simulink model "mysldemo_2counters"  (R2014a)
settings: Solver=FixedStepDiscrete  StartTime=0.0  StopTime=2.5  FixedStep=.01  RelTol=1e-3  AbsTol=1e-6
undefined symbols (not defined in the file): sigbuilder_block
Description:
  | Counters Using Conditionally Executed Subsystems
  | 
  | This demonstration uses counter circuits to contrast the execution of blocks in enabled
  | subsystems and triggered subsystems for the same control signal. After running the
  | simulation, the scope shows three plots.
  | 
  | The first of these plots shows the control signal which is the output of the discrete
  | pulse generator.
  | 
  | The second plot shows the output of the counter circuit in the enabled subsystem.
  | The counter increments while the subsystem is enabled and then holds its output when
  | the subsystem is disabled. The counter resets to zero when the subsystem is re-enabled
  | because the enable port was configured to reset states when enabling.
  | 
  | The third plot shows the output of the counter circuit in the triggered subsystem. The
  | counter increments every rising edge of the control signal.
  | 
  | The signals are shown in a Signal Viewer scope that does not require a scope block to
  | be put into the block diagram.  Instead, the "glasses" icon notation on the ports show
  | that a Signal Viewer is attached.  Double click on the glasses to make the Signal
  | Viewer appear if it is hidden.
settings Model: RecordCoverage=on  CovMetricSettings=de  CovHTMLOptions=-aTS=1 -bRG=1 -bTC=1 -hTR=0 -nFC=0 -scm=1 -bcm=1 -xEv=0  CovHtmlReporting=off  CovForceBlockReductionOff=off  covSaveCumulativeToWorkspaceVar=off  CovSaveSingleToWorkspaceVar=off  CovCumulativeReport=on  CovReportOnPause=off  ExtModeTrigMode=oneshot  ExtModeArmWhenConnect=off  ExtModeAutoUpdateStatusClock=off  Creator=The MathWorks Inc.  LastModifiedBy=gxnuhuang
settings DataIOCC: LimitDataPoints=off  SaveFormat=StructureWithTime  DSMLogging=off  InspectSignalLogs=on  ReturnWorkspaceOutputs=on
settings OptimizationCC: BlockReduction=off  BooleanDataType=off  ExpressionDepthLimit=2147483647  InitFltsAndDblsToZero=on  BufferReusableBoundary=off
settings DebuggingCC: SaveWithParameterizedLinksMsg=none  UnderspecifiedInitializationDetection=Classic  SignalResolutionControl=TryResolveAllWithWarning  SolverPrmCheckMsg=none  MultiTaskDSMMsg=warning  MultiTaskCondExecSysMsg=none  FcnCallInpInsideContextMsg=UseLocalSettings  BusObjectLabelMismatch=none  StateNameClashWarn=warning
settings HardwareCC: TargetUnknown=on
settings RTWCC: IncludeERTFirstTime=on
settings GRTTargetCC: TargetFcnLib=ansi_tfl_tmw.mat  CombineOutputUpdateFcns=off  GRTInterface=on

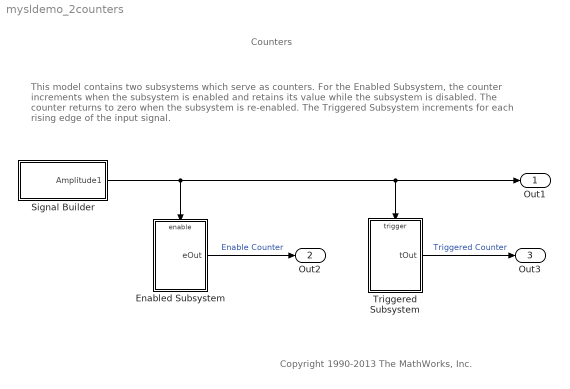
== system mysldemo_2counters ==
  note: Counters
  note: Copyright 1990-2013 The MathWorks, Inc.
  note: This model contains two subsystems which serve as counters. For the Enabled Subsystem, the counter
      | increments when the subsystem is enabled and retains its value while the subsystem is disabled.
      | The counter returns to zero when the subsystem is re-enabled.  The Triggered Subsystem increments
      | for each rising edge of the input signal.
  Enabled Subsystem : Subsystem  TreatAsAtomicUnit=on
  Signal Builder : Subsystem  Tag=STV Subsys  LoadFcn=sigbuilder_block('load');  StartFcn=sigbuilder_block('start');  StopFcn=sigbuilder_block('stop');  ClipboardFcn=sigbuilder_block('clipboard');  mask(Sigbuilder block){}
      mask help: Create and generate interchangeable groups of signals whose waveforms are piecewise linear.
      mask init:
      | if ~strcmp(get_param(bdroot(gcbh),'SimulationStatus'),'stopped') tuvar = sigbuilder_block('maskInit'); end
      settings: CopyFcn=sigbuilder_block('copy');  DeleteFcn=sigbuilder_block('delete');  ModelCloseFcn=sigbuilder_block('modelClose');  PreSaveFcn=sigbuilder_block('preSave');  PauseFcn=sigbuilder_block('pause')  ContinueFcn=sigbuilder_block('continue')  NameChangeFcn=sigbuilder_block('namechange');  OpenFcn=sigbuilder_block('open',[192.75 138 550.5 399.75 ]);  CloseFcn=sigbuilder_block('close');
      mask Display: plot(0,0,100,100,[10,10,40,40,10],[80,20,20,80,80],[40,10],[50,50], [40,27,10],[65,72,56],[40,25,25,10],[28,28,43,43]);
  Triggered Subsystem : Subsystem  TreatAsAtomicUnit=on
  Out1 : Outport
  Out2 : Outport  Port=2
  Out3 : Outport  Port=3
  wires:
  Enabled Subsystem/1(eOut) -> Out2/1  "Enable Counter"
  Triggered Subsystem/1(tOut) -> Out3/1  "Triggered Counter"
  Signal Builder/1(Amplitude1) -> Enabled Subsystem/Enable, Triggered Subsystem/Trigger, Out1/1

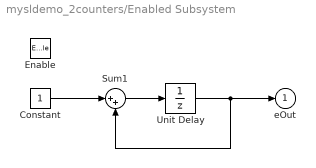
== system mysldemo_2counters/Enabled Subsystem ==
  Enable : EnablePort  StatesWhenEnabling=reset
  Constant : Constant
  Sum1 : Sum  Inputs=|++  SaturateOnIntegerOverflow=on  InputSameDT=on  OutDataTypeStr=Inherit: Same as first input
  Unit Delay : UnitDelay  SampleTime=.01
  eOut : Outport  InitialOutput=0
  wires:
  Sum1/1 -> Unit Delay/1
  Constant/1 -> Sum1/1
  Unit Delay/1 -> eOut/1, Sum1/2

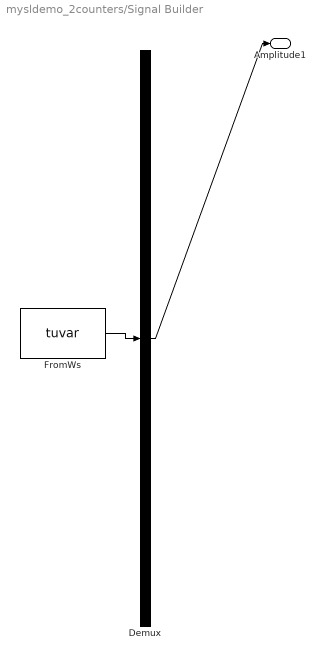
== system mysldemo_2counters/Signal Builder ==
  Demux : Demux  Tag=STV Demux  Outputs=1
  FromWs : FromWorkspace  Tag=STV FromWs  VariableName=tuvar  SampleTime=0
      SigBuilderData=|
      | common.afterFinalStr = 'Extrapolate'
      | common.sampleTime = 0
      | dataSet(1).timeRange = [0 10]
      | dataSet(1).name = 'Impulse Input'
      | dataSet(2).timeRange = [0 10]
      | dataSet(2).name = 'Ramp Input'
      | sbobj.Groups(1).Name = 'Impulse Input'
      | sbobj.Groups(1).Signals.Name = 'Amplitude1'
      | sbobj.Groups(1).Signals.XData = [0 0.2 0.2 0.4 0.4 0.6 0.6 0.8 0.8 1 1 1.2 1.2 1.4 1.4 1.6 1.6 1.8 1.8 2 2 10]
      | sbobj.Groups(1).Signals.YData = [0 0 1 1 0 0 1 1 0 0 1 1 0 0 1 1 0 0 1 1 0 0]
      | sbobj.Groups(2).Name = 'Ramp Input'
      | sbobj.Groups(2).Signals.Name = 'Amplitude1'
      | sbobj.Groups(2).Signals.XData = [0 0.2 0.4 0.6 0.8 1 1.2 1.4 1.6 1.8 2 10]
      | sbobj.Groups(2).Signals.YData = [0 1 0 1 0 1 0 1 0 1 0 0]
  Amplitude1 : Outport  Tag=STV Outport
  wires:
  FromWs/1 -> Demux/1
  Demux/1 -> Amplitude1/1

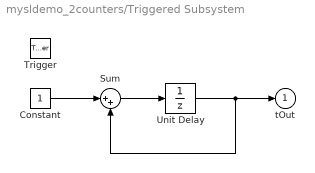
== system mysldemo_2counters/Triggered Subsystem ==
  Trigger : TriggerPort
  Constant : Constant
  Sum : Sum  Inputs=|++  SaturateOnIntegerOverflow=on  InputSameDT=on  OutDataTypeStr=Inherit: Same as first input
  Unit Delay : UnitDelay  SampleTime=-1
  tOut : Outport  InitialOutput=0
  wires:
  Sum/1 -> Unit Delay/1
  Constant/1 -> Sum/1
  Unit Delay/1 -> tOut/1, Sum/2
